simulink model "Calculator"  (R2021a)
settings: Solver=FixedStepDiscrete  StartTime=0.0  StopTime=10.0  RelTol=1e-3  EnableMultiTasking=on
settings Model: Creator=alyma  LastModifiedBy=alyma
settings DataIOCC: ReturnWorkspaceOutputs=off
settings OptimizationCC: DefaultParameterBehavior=Inlined  InlineInvariantSignals=on  EnableMemcpy=off  LifeSpan=1  EfficientTunableParamExpr=on
settings DebuggingCC: UnderspecifiedInitializationDetection=Classic  MergeDetectMultiDrivingBlocksExec=none  SFMachineParentedDataDiag=warning  ArithmeticOperatorsInVariantConditions=warning
settings ModelReferenceCC: PropagateSignalLabelsOutOfModel=off
settings SFSimCC: MATLABDynamicMemAlloc=off  CustomCodeUndefinedFunction=UseInterfaceOnly
settings RTWCC: SystemTargetFile=ert.tlc  GenCodeOnly=on  TemplateMakefile=ert_default_tmf  GenerateReport=on  IncludeHyperlinkInReport=on  LaunchReport=on  GenerateTraceInfo=on  GenerateTraceReport=on  GenerateTraceReportSl=on  GenerateTraceReportSf=on  GenerateTraceReportEml=on
settings CodeAppCC: ForceParamTrailComments=on  IgnoreCustomStorageClasses=off  OperatorAnnotations=on  SimulinkDataObjDesc=on  SFDataObjDesc=on  MATLABFcnDesc=on  InsertBlockDesc=on  StateflowObjectComments=on  MATLABSourceComments=on
settings ERTTargetCC: MultiwordLength=2048  GenerateSampleERTMain=on  InlinedParameterPlacement=NonHierarchical  ERTCustomFileTemplate=example_file_process.tlc

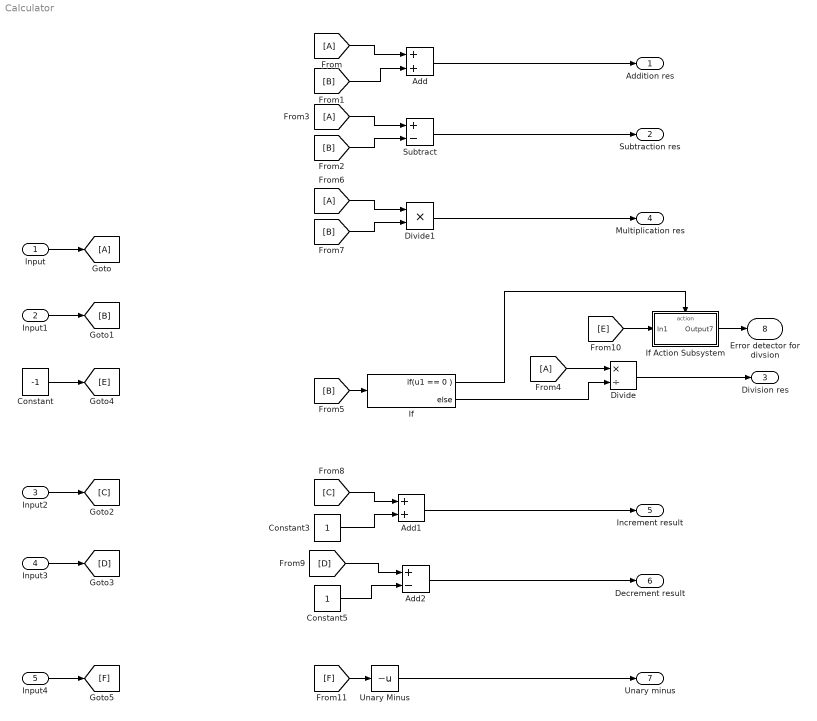
== system Calculator ==
  Input : Inport
  Input1 : Inport  Port=2
  Input2 : Inport  Port=3
  Input3 : Inport  Port=4
  Input4 : Inport  Port=5
  Add : Sum
  Add1 : Sum
  Add2 : Sum  Inputs=+-
  Constant : Constant  Value=-1
  Constant3 : Constant
  Constant5 : Constant
  Divide : Product  Inputs=*/
  Divide1 : Product  Inputs=**
  If : If  IfExpression=u1 == 0
  If Action Subsystem : Subsystem  TreatAsAtomicUnit=on
  Subtract : Sum  Inputs=+-
  Unary Minus : UnaryMinus
  Addition res : Outport
  Subtraction res : Outport  Port=2
  Division res : Outport  Port=3
  Multiplication res : Outport  Port=4
  Increment result : Outport  Port=5
  Decrement result : Outport  Port=6
  Unary minus : Outport  Port=7
  Error detector for divsion : Outport  Port=8
  wires:
  [A] -> Add/1
  [B] -> Add/2
  [A] -> Subtract/1
  [B] -> Subtract/2
  [A] -> Divide1/1
  [B] -> Divide1/2
  Add/1 -> Addition res/1
  Subtract/1 -> Subtraction res/1
  Divide/1 -> Division res/1
  Divide1/1 -> Multiplication res/1
  Input2/1 -> [C]
  [C] -> Add1/1
  Constant3/1 -> Add1/2
  Add1/1 -> Increment result/1
  Input3/1 -> [D]
  Constant5/1 -> Add2/2
  [D] -> Add2/1
  Unary Minus/1 -> Unary minus/1
  Add2/1 -> Decrement result/1
  Input/1 -> [A]
  Input1/1 -> [B]
  [A] -> Divide/1
  [B] -> If/1
  If/2 -> Divide/2
  If/1 -> If Action Subsystem/Action
  [E] -> If Action Subsystem/1(In1)
  Constant/1 -> [E]
  If Action Subsystem/1(Output7) -> Error detector for divsion/1
  [F] -> Unary Minus/1
  Input4/1 -> [F]

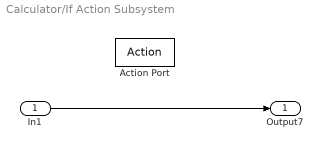
== system Calculator/If Action Subsystem ==
  In1 : Inport
  Action Port : ActionPort  ActionPortLabel=if(u1 == 0 )
  Output7 : Outport
  wires:
  In1/1 -> Output7/1
